simulink model "s1"  (R2015b)
settings: Solver=ode4  StartTime=0.0  StopTime=0.2  RelTol=1e-3
values from neighbouring files (symbols this model uses):
  delta_z = L/(N-1)    (= 7.5)    [assignment.m]
  dpdz = 80    [assignment.m]
  Q0 = 16.7    [assignment.m]
  ro = 15    [assignment.m]
  s0 = 1.2    [assignment.m]
  v = 0.035    [assignment.m]
settings Model: Creator=eBrand  LastModifiedBy=eBrand

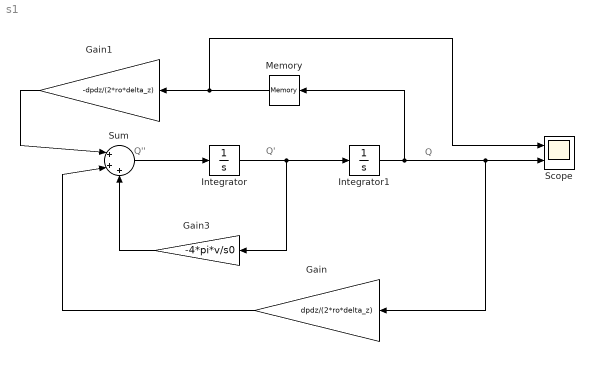
== system s1 ==
  note: Q''
  note: Q
  note: Q'
  Gain : Gain  Gain=dpdz/(2*ro*delta_z)
  Gain1 : Gain  Gain=-dpdz/(2*ro*delta_z)
  Gain3 : Gain  Gain=-4*pi*v/s0
  Integrator : Integrator
  Integrator1 : Integrator
  Memory : Memory  X0=Q0
  Scope : Scope  NumInputPorts=2
  Sum : Sum  Inputs=|+++
  wires:
  Integrator/1 -> Gain3/1, Integrator1/1
  Sum/1 -> Integrator/1
  Integrator1/1 -> Memory/1, Gain/1, Scope/2
  Gain/1 -> Sum/2
  Gain3/1 -> Sum/3
  Gain1/1 -> Sum/1
  Memory/1 -> Scope/1, Gain1/1
